simulink model "MRAC_Output_Measurement"  (R2016b)
settings: Solver=VariableStepAuto  StartTime=0.0  StopTime=10.0  RelTol=1e-3
undefined symbols (not defined in the file or in its folder): sigbuilder_block
settings Model: Creator=Niels  LastModifiedBy=Niels

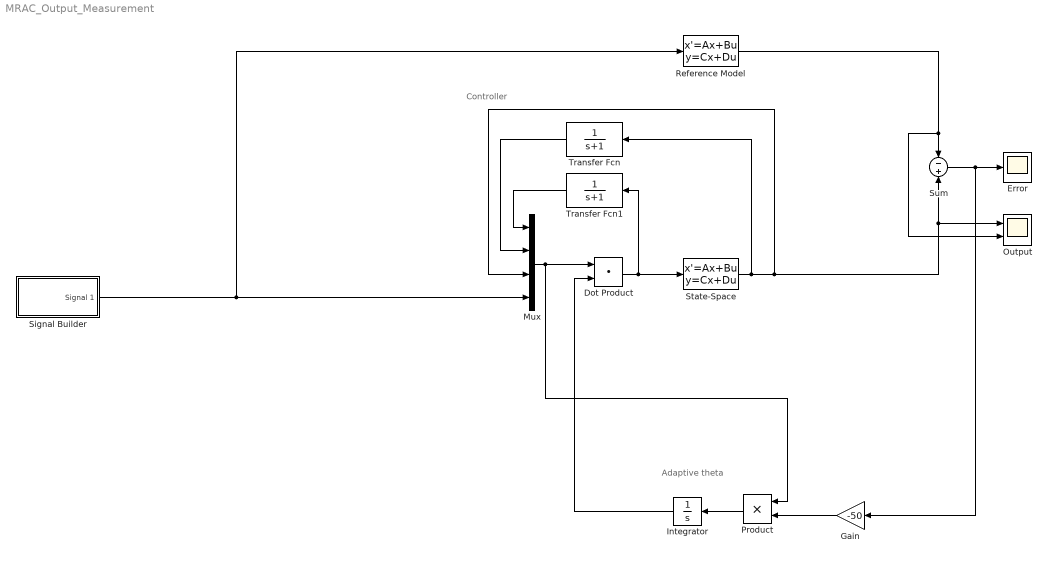
== system MRAC_Output_Measurement ==
  note: Adaptive theta
  note: Controller
  Dot Product : DotProduct  InputSameDT=on  OutDataTypeStr=Inherit: Inherit via internal rule
  Error : Scope
  Gain : Gain  Gain=-50
  Integrator : Integrator
  Mux : Mux
  Output : Scope  NumInputPorts=2
  Product : Product
  "Reference Model " : StateSpace  A=[-15 -50;1 0]  B=[1;0]  C=[1 50]  D=0  X0=0
  Signal Builder : Subsystem  Tag=STV Subsys  LoadFcn=sigbuilder_block('load');  StartFcn=sigbuilder_block('start');  StopFcn=sigbuilder_block('stop');  ClipboardFcn=sigbuilder_block('clipboard');  mask(Sigbuilder block){tuvar=[0:10]}
      mask help: Simulink:masks:SigbuilderBlock_MD
      mask init:
      | if ~strcmp(get_param(bdroot(gcbh),'SimulationStatus'),'stopped') tuvar = sigbuilder_block('maskInit'); end
      settings: CopyFcn=sigbuilder_block('copy');  DeleteFcn=sigbuilder_block('delete');  ModelCloseFcn=sigbuilder_block('modelClose');  PreSaveFcn=sigbuilder_block('preSave');  PauseFcn=sigbuilder_block('pause');  ContinueFcn=sigbuilder_block('continue');  NameChangeFcn=sigbuilder_block('namechange');  OpenFcn=sigbuilder_block('open',[437.6 199.2 550.4 400 ]);  CloseFcn=sigbuilder_block('close');
      mask Display: plot(0, 0, 100, 100,[2, 2, 32, 32, 2], [68, 8, 8, 68, 68],[32, 2], [38, 38], [32, 19, 2],[53, 60, 44], [32, 17, 17, 2],[16, 16, 31, 31]);txt = getActiveGroup(gcbh);text(2, 100, txt,'verticalAlignment', 'top');
  State-Space : StateSpace  A=[-0.75 -2.5;1 0]  B=[1;0]  C=[1 1.5]  D=[0]  X0=[1;-1]
  Sum : Sum  Inputs=-|+
  Transfer Fcn : TransferFcn  Denominator=[1 1]
  Transfer Fcn1 : TransferFcn  Denominator=[1 1]
  wires:
  Signal Builder/1(Signal 1) -> Mux/4, "Reference Model "/1
  Dot Product/1 -> Transfer Fcn1/1, State-Space/1
  Mux/1 -> Product/1, Dot Product/1
  "Reference Model "/1 -> Output/2, Sum/1
  State-Space/1 -> Transfer Fcn/1, Mux/3, Sum/2, Output/1
  Sum/1 -> Gain/1, Error/1
  Transfer Fcn/1 -> Mux/2
  Transfer Fcn1/1 -> Mux/1
  Gain/1 -> Product/2
  Product/1 -> Integrator/1
  Integrator/1 -> Dot Product/2

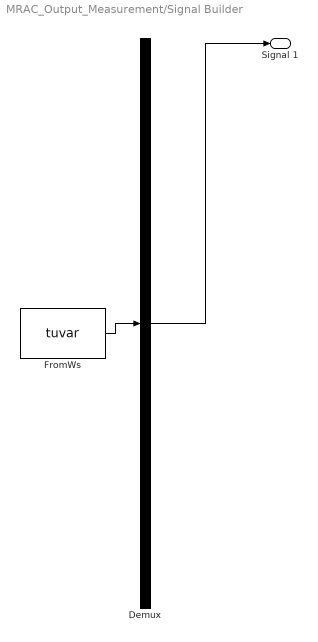
== system MRAC_Output_Measurement/Signal Builder ==
  Demux : Demux  Tag=STV Demux  Outputs=1
  FromWs : FromWorkspace  Tag=STV FromWs  VariableName=tuvar  SampleTime=0
      SigBuilderData=|
      | common.afterFinalStr = 'Extrapolate'
      | common.sampleTime = 0
      | dataSet.timeRange = [0 10]
      | dataSet.name = 'Group 1'
      | sbobj.Groups.Name = 'Group 1'
      | sbobj.Groups.Signals.Name = 'Signal 1'
      | sbobj.Groups.Signals.XData = [0 1 1 10]
      | sbobj.Groups.Signals.YData = [0 0 1 1]
  Signal 1 : Outport  Tag=STV Outport
  wires:
  Demux/1 -> Signal 1/1
  FromWs/1 -> Demux/1
